simulink model "SimControl_new"  (R2021b)
settings: Solver=ode45  StartTime=0.0  StopTime=inf  RelTol=1e-3
libraries: slpidlib x3, etargetslib x2, dspnetwork x2, sldrtlib x2, simulink_extras x1
settings Model: Creator=Flight Test Lab  LastModifiedBy=jakub
settings SolverCC: AlgebraicLoopSolver=TrustRegion
settings DataIOCC: SaveFormat=StructureWithTime  ReturnWorkspaceOutputs=off
settings OptimizationCC: LifeSpan=inf
settings DebuggingCC: SFExecutionAtInitializationDiag=none  SFMachineParentedDataDiag=warning  ArithmeticOperatorsInVariantConditions=warning
settings HardwareCC: ProdBitPerSizeT=32  ProdBitPerPtrDiffT=32  ProdWordSize=32  ProdHWDeviceType=Specified
settings SFSimCC: SimUseLocalCustomCode=off  CustomCodeUndefinedFunction=UseInterfaceOnly
settings RTWCC: RTWUseLocalCustomCode=off
settings CodeAppCC: StateflowObjectComments=on

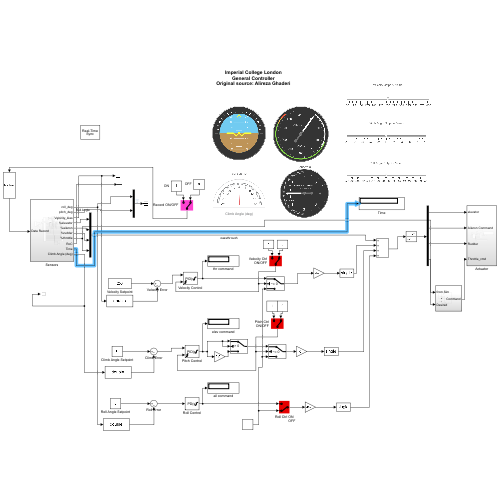
[thumbnail: Simulink's stored preview of the top-level diagram]
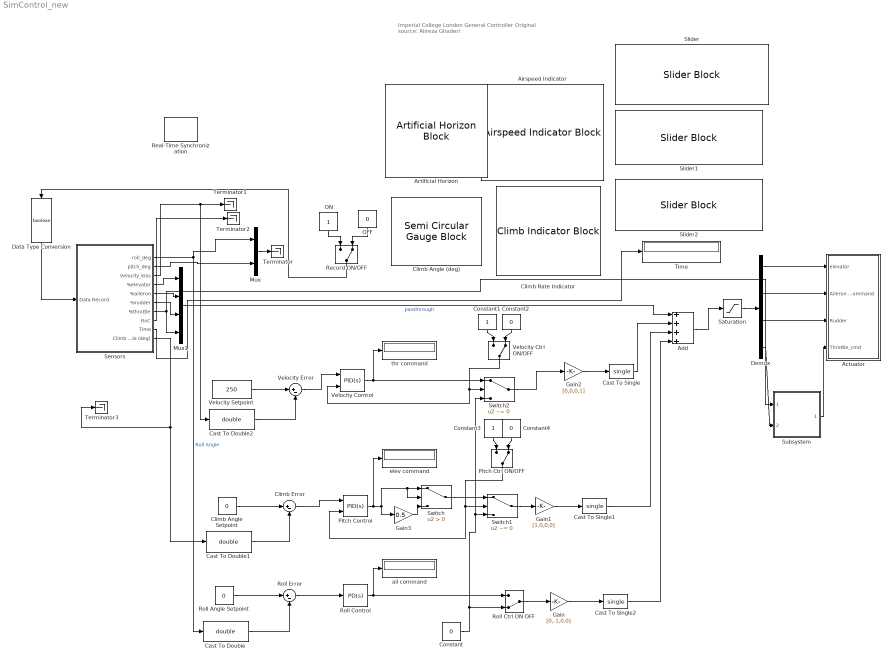
== system SimControl_new ==
  note: Imperial College London
      | General Controller
      | Original source: Alireza Ghaderi
  Actuator : Subsystem
  Add : Sum  Inputs=++++
  Airspeed Indicator : AirspeedIndicatorBlock  LabelPosition=Hide  ScaleMin=0  ScaleMax=450
  Artificial Horizon : ArtificialHorizonBlock  LabelPosition=Hide
  Cast To Double : DataTypeConversion  OutDataTypeStr=double
  Cast To Double1 : DataTypeConversion  OutDataTypeStr=double
  Cast To Double2 : DataTypeConversion  OutDataTypeStr=double
  Cast To Single : DataTypeConversion  OutDataTypeStr=single
  Cast To Single1 : DataTypeConversion  OutDataTypeStr=single
  Cast To Single2 : DataTypeConversion  OutDataTypeStr=single
  Climb Angle (deg) : SemiCircularGaugeBlock  ScaleMin=-20  ScaleMax=20
  Climb Angle Setpoint : Constant  Value=0
  Climb Error : Sum  Inputs=|+-
  Climb Rate Indicator : ClimbIndicatorBlock
  Constant : Constant  Value=0
  Constant1 : Constant
  Constant2 : Constant  Value=0
  Constant3 : Constant
  Constant4 : Constant  Value=0
  Data Type Conversion : DataTypeConversion  OutDataTypeStr=boolean
  Demux : Demux
  Gain : Gain  Gain=[0,-1,0,0]
  Gain1 : Gain  Gain=[1,0,0,0]
  Gain2 : Gain  Gain=[0,0,0,1]
  Gain3 : Gain  Gain=0.5
  Mux : Mux  Inputs=2
  Mux1 : Mux
  OFF : Constant  Value=0
  ON : Constant
  Pitch Control : slpidlib/PID Controller  Controller=PID  Form=Parallel  TimeDomain=Continuous-time  UseExternalTs=off  SampleTime=-1  IntegratorMethod=Forward Euler  FilterMethod=Forward Euler  ControllerParametersSource=internal  P=0.15  I=0.04  D=0.05  UseFilter=on  N=100  TunerSelectOption=Transfer Function Based (PID Tuner App)  InitialConditionSource=internal  InitialConditionForIntegrator=0  InitialConditionForFilter=0  DifferentiatorICPrevScaledInput=0  ExternalReset=rising  TrackingMode=off  Kt=1  LimitOutput=on  SatLimitsSource=internal  UpperSaturationLimit=1  LowerSaturationLimit=-2  LinearizeAsGain=on  AntiWindupMode=clamping  Kb=1  POutMin=[]  POutMax=[]  IOutMin=[]  IOutMax=[]  DOutMin=[]  DOutMax=[]  NOutMin=[]  NOutMax=[]  SumOutMin=[]  SumOutMax=[]  SaturationOutMin=[]  SaturationOutMax=[]  PParamMin=[]  PParamMax=[]  IParamMin=[]  IParamMax=[]  DParamMin=[]  DParamMax=[]  NParamMin=[]  NParamMax=[]  KbParamMin=[]  KbParamMax=[]  KtParamMin=[]  KtParamMax=[]  KbOutMin=[]  KbOutMax=[]  KtOutMin=[]  KtOutMax=[]  IntegratorOutMin=[]  IntegratorOutMax=[]  FilterOutMin=[]  FilterOutMax=[]  SumI1OutMin=[]  SumI1OutMax=[]  SumI2OutMin=[]  SumI2OutMax=[]  SumI3OutMin=[]  SumI3OutMax=[]  SumI4OutMin=[]  SumI4OutMax=[]  SumDOutMin=[]  SumDOutMax=[]  DifferentiatorOutMin=[]  DifferentiatorOutMax=[]  FilterDiffOutCoefMin=[]  FilterDiffOutCoefMax=[]  ReciprocalOutMin=[]  ReciprocalOutMax=[]  SumDenOutMin=[]  SumDenOutMax=[]  SumNumOutMin=[]  SumNumOutMax=[]  DivideOutMin=[]  DivideOutMax=[]  UdiffTsProdOutMin=[]  UdiffTsProdOutMax=[]  NTsProdOutMin=[]  NTsProdOutMax=[]  UintegralTsProdOutMin=[]  UintegralTsProdOutMax=[]  UngainTsProdOutMin=[]  UngainTsProdOutMax=[]  IntegratorContinuousStateAttributes=''  IntegratorStateMustResolveToSignalObject=off  IntegratorRTWStateStorageClass=Auto  FilterContinuousStateAttributes=''  FilterStateMustResolveToSignalObject=off  FilterRTWStateStorageClass=Auto  ParallelPVariant=InternalParameters  IdealPVariant=Disabled  IVariant=InternalParameters  DVariant=InternalParameters  IntegratorVariant=Continuous  SatVariant=Enabled  AWVariant=ContClampingParallel  PCopyVariant=Disabled  TRVariant=Disabled  FdbkBlocksVariant=Forward  IdealPFdbkVariant=Disabled  SatFdbkVariant=Disabled  DerivativeFilterVariant=ContFilter  NVariant=InternalParameters  NCopyVariant=Disabled  FilterICVariant=InternalICsFilter  IntegratorICVariant=InternalICs  ExternalResetVariant=ExternalReset  TRSumVariant=Passthrough  SumFdbkVariant=Disabled  SumVariant=Sum_PID  TsampFilterVariant=InternalTs  TsampNgainVariant=Passthrough  TsampIntegralVariant=Passthrough  ExternalSaturationOutDataTypeStr=Inherit: Same as second input
  Pitch Ctrl ON/OFF : ManualSwitch  CurrentSetting=0
  Real-Time Synchronization : sldrtlib/Real-Time Synchronization  SampleTime=0.05  MaxMissedTicks=100  ShowMissedTicks=off  YieldWhenWaiting=off
  Record ON/OFF : ManualSwitch  CurrentSetting=0
  Roll Angle Setpoint : Constant  Value=0
  Roll Control : slpidlib/PID Controller  Controller=PD  Form=Parallel  TimeDomain=Continuous-time  UseExternalTs=off  SampleTime=-1  IntegratorMethod=Forward Euler  FilterMethod=Forward Euler  ControllerParametersSource=internal  P=-0.7  I=1  D=-0.05  UseFilter=on  N=100  TunerSelectOption=Transfer Function Based (PID Tuner App)  InitialConditionSource=internal  InitialConditionForIntegrator=0  InitialConditionForFilter=0  DifferentiatorICPrevScaledInput=0  ExternalReset=none  TrackingMode=off  Kt=1  LimitOutput=on  SatLimitsSource=internal  UpperSaturationLimit=1  LowerSaturationLimit=-1  LinearizeAsGain=on  AntiWindupMode=none  Kb=1  POutMin=[]  POutMax=[]  IOutMin=[]  IOutMax=[]  DOutMin=[]  DOutMax=[]  NOutMin=[]  NOutMax=[]  SumOutMin=[]  SumOutMax=[]  SaturationOutMin=[]  SaturationOutMax=[]  PParamMin=[]  PParamMax=[]  IParamMin=[]  IParamMax=[]  DParamMin=[]  DParamMax=[]  NParamMin=[]  NParamMax=[]  KbParamMin=[]  KbParamMax=[]  KtParamMin=[]  KtParamMax=[]  KbOutMin=[]  KbOutMax=[]  KtOutMin=[]  KtOutMax=[]  IntegratorOutMin=[]  IntegratorOutMax=[]  FilterOutMin=[]  FilterOutMax=[]  SumI1OutMin=[]  SumI1OutMax=[]  SumI2OutMin=[]  SumI2OutMax=[]  SumI3OutMin=[]  SumI3OutMax=[]  SumI4OutMin=[]  SumI4OutMax=[]  SumDOutMin=[]  SumDOutMax=[]  DifferentiatorOutMin=[]  DifferentiatorOutMax=[]  FilterDiffOutCoefMin=[]  FilterDiffOutCoefMax=[]  ReciprocalOutMin=[]  ReciprocalOutMax=[]  SumDenOutMin=[]  SumDenOutMax=[]  SumNumOutMin=[]  SumNumOutMax=[]  DivideOutMin=[]  DivideOutMax=[]  UdiffTsProdOutMin=[]  UdiffTsProdOutMax=[]  NTsProdOutMin=[]  NTsProdOutMax=[]  UintegralTsProdOutMin=[]  UintegralTsProdOutMax=[]  UngainTsProdOutMin=[]  UngainTsProdOutMax=[]  IntegratorContinuousStateAttributes=''  IntegratorStateMustResolveToSignalObject=off  IntegratorRTWStateStorageClass=Auto  FilterContinuousStateAttributes=''  FilterStateMustResolveToSignalObject=off  FilterRTWStateStorageClass=Auto  ParallelPVariant=InternalParameters  IdealPVariant=Disabled  IVariant=Disabled  DVariant=InternalParameters  IntegratorVariant=Disabled  SatVariant=Enabled  AWVariant=Disabled  PCopyVariant=Disabled  TRVariant=Disabled  FdbkBlocksVariant=Forward  IdealPFdbkVariant=Disabled  SatFdbkVariant=Disabled  DerivativeFilterVariant=ContFilter  NVariant=InternalParameters  NCopyVariant=Disabled  FilterICVariant=InternalICsFilter  IntegratorICVariant=Disabled  ExternalResetVariant=Disabled  TRSumVariant=Passthrough  SumFdbkVariant=Disabled  SumVariant=Sum_PD  TsampFilterVariant=InternalTs  TsampNgainVariant=Passthrough  TsampIntegralVariant=Disabled_SignalSpec  ExternalSaturationOutDataTypeStr=Inherit: Same as second input
  Roll Ctrl ON OFF : ManualSwitch  CurrentSetting=0
  Roll Error : Sum  Inputs=|+-
  Saturation : Saturate  UpperLimit=[1,1,1,1]  LowerLimit=[-1,-1,-1,0]
  Sensors : Subsystem
  Slider : SliderBlock  ScaleMin=100  ScaleMax=400
  Slider1 : SliderBlock  ScaleMin=-10  ScaleMax=10  TickInterval=2
  Slider2 : SliderBlock  ScaleMin=-45  ScaleMax=45
  Subsystem : Subsystem
  Switch : Switch  Criteria=u2 > Threshold
  Switch1 : Switch  Criteria=u2 ~= 0
  Switch2 : Switch  Criteria=u2 ~= 0
  Terminator{,1..3} (4 alike) : Terminator
  Time : Display
  Velocity Control : slpidlib/PID Controller  Controller=PID  Form=Parallel  TimeDomain=Continuous-time  UseExternalTs=off  SampleTime=-1  IntegratorMethod=Forward Euler  FilterMethod=Forward Euler  ControllerParametersSource=internal  P=3  I=0.1  D=0.2  UseFilter=on  N=100  TunerSelectOption=Transfer Function Based (PID Tuner App)  InitialConditionSource=internal  InitialConditionForIntegrator=0  InitialConditionForFilter=0  DifferentiatorICPrevScaledInput=0  ExternalReset=rising  TrackingMode=off  Kt=1  LimitOutput=on  SatLimitsSource=internal  UpperSaturationLimit=1  LowerSaturationLimit=-1  LinearizeAsGain=on  AntiWindupMode=clamping  Kb=1  POutMin=[]  POutMax=[]  IOutMin=[]  IOutMax=[]  DOutMin=[]  DOutMax=[]  NOutMin=[]  NOutMax=[]  SumOutMin=[]  SumOutMax=[]  SaturationOutMin=[]  SaturationOutMax=[]  PParamMin=[]  PParamMax=[]  IParamMin=[]  IParamMax=[]  DParamMin=[]  DParamMax=[]  NParamMin=[]  NParamMax=[]  KbParamMin=[]  KbParamMax=[]  KtParamMin=[]  KtParamMax=[]  KbOutMin=[]  KbOutMax=[]  KtOutMin=[]  KtOutMax=[]  IntegratorOutMin=[]  IntegratorOutMax=[]  FilterOutMin=[]  FilterOutMax=[]  SumI1OutMin=[]  SumI1OutMax=[]  SumI2OutMin=[]  SumI2OutMax=[]  SumI3OutMin=[]  SumI3OutMax=[]  SumI4OutMin=[]  SumI4OutMax=[]  SumDOutMin=[]  SumDOutMax=[]  DifferentiatorOutMin=[]  DifferentiatorOutMax=[]  FilterDiffOutCoefMin=[]  FilterDiffOutCoefMax=[]  ReciprocalOutMin=[]  ReciprocalOutMax=[]  SumDenOutMin=[]  SumDenOutMax=[]  SumNumOutMin=[]  SumNumOutMax=[]  DivideOutMin=[]  DivideOutMax=[]  UdiffTsProdOutMin=[]  UdiffTsProdOutMax=[]  NTsProdOutMin=[]  NTsProdOutMax=[]  UintegralTsProdOutMin=[]  UintegralTsProdOutMax=[]  UngainTsProdOutMin=[]  UngainTsProdOutMax=[]  IntegratorContinuousStateAttributes=''  IntegratorStateMustResolveToSignalObject=off  IntegratorRTWStateStorageClass=Auto  FilterContinuousStateAttributes=''  FilterStateMustResolveToSignalObject=off  FilterRTWStateStorageClass=Auto  ParallelPVariant=InternalParameters  IdealPVariant=Disabled  IVariant=InternalParameters  DVariant=InternalParameters  IntegratorVariant=Continuous  SatVariant=Enabled  AWVariant=ContClampingParallel  PCopyVariant=Disabled  TRVariant=Disabled  FdbkBlocksVariant=Forward  IdealPFdbkVariant=Disabled  SatFdbkVariant=Disabled  DerivativeFilterVariant=ContFilter  NVariant=InternalParameters  NCopyVariant=Disabled  FilterICVariant=InternalICsFilter  IntegratorICVariant=InternalICs  ExternalResetVariant=ExternalReset  TRSumVariant=Passthrough  SumFdbkVariant=Disabled  SumVariant=Sum_PID  TsampFilterVariant=InternalTs  TsampNgainVariant=Passthrough  TsampIntegralVariant=Passthrough  ExternalSaturationOutDataTypeStr=Inherit: Same as second input
  Velocity Ctrl ON/OFF : ManualSwitch  CurrentSetting=0
  Velocity Error : Sum  Inputs=|+-
  Velocity Setpoint : Constant  Value=250
  ail command : Display
  elev command : Display
  thr command : Display
  wires:
  Sensors/1(roll_deg) -> Mux/1, Cast To Double/1  "Roll Angle"
  Sensors/2(pitch_deg) -> Mux/2
  Mux/1 -> Terminator/1
  Sensors/4(%elevator) -> Mux1/1
  Sensors/5(%aileron) -> Mux1/2
  Sensors/6(%rudder) -> Mux1/3
  Sensors/7(%throttle) -> Mux1/4, Subsystem/1(from Sim)
  Demux/1 -> Actuator/1(elevator)
  Demux/2 -> Actuator/2(Aileron Command)
  Demux/3 -> Actuator/3("Rudder ")
  Sensors/3(Velocity_kias) -> Terminator1/1, Cast To Double2/1
  Mux1/1 -> Add/1  "passthrough"
  Roll Angle Setpoint/1 -> Roll Error/1
  Climb Angle Setpoint/1 -> Climb Error/1
  Velocity Setpoint/1 -> Velocity Error/1
  Roll Ctrl ON OFF/1 -> Gain/1
  Gain/1 -> Cast To Single2/1
  Constant/1 -> Roll Ctrl ON OFF/2, Switch2/3, Switch1/3
  Roll Error/1 -> Roll Control/1
  Roll Control/1 -> ail command/1, Roll Ctrl ON OFF/1
  Cast To Double/1 -> Roll Error/2
  Cast To Double1/1 -> Climb Error/2
  Cast To Double2/1 -> Velocity Error/2
  Velocity Error/1 -> Velocity Control/1
  Climb Error/1 -> Pitch Control/1
  Gain1/1 -> Cast To Single1/1
  Switch1/1 -> Gain1/1
  Gain3/1 -> Switch/3
  Pitch Control/1 -> elev command/1, Gain3/1, Switch/1, Switch/2
  Switch/1 -> Switch1/1
  Add/1 -> Saturation/1
  Saturation/1 -> Demux/1
  Velocity Control/1 -> thr command/1, Switch2/1
  Cast To Single/1 -> Add/2
  Cast To Single1/1 -> Add/3
  Cast To Single2/1 -> Add/4
  Record ON/OFF/1 -> Data Type Conversion/1
  OFF/1 -> Record ON/OFF/2
  ON/1 -> Record ON/OFF/1
  Data Type Conversion/1 -> Sensors/1(Data Record)
  Sensors/8(RoC) -> Terminator2/1
  Sensors/9(Time) -> Time/1
  Sensors/10(Climb Angle (deg)) -> Terminator3/1, Cast To Double1/1
  Velocity Ctrl ON/OFF/1 -> Switch2/2, Velocity Control/2
  Pitch Ctrl ON/OFF/1 -> Pitch Control/2, Switch1/2
  Constant1/1 -> Velocity Ctrl ON/OFF/1
  Constant2/1 -> Velocity Ctrl ON/OFF/2
  Constant3/1 -> Pitch Ctrl ON/OFF/1
  Constant4/1 -> Pitch Ctrl ON/OFF/2
  Subsystem/1(Command) -> Actuator/4(Throttle_cmd)
  Switch2/1 -> Gain2/1
  Gain2/1 -> Cast To Single/1
  Demux/4 -> Subsystem/2(Desired)

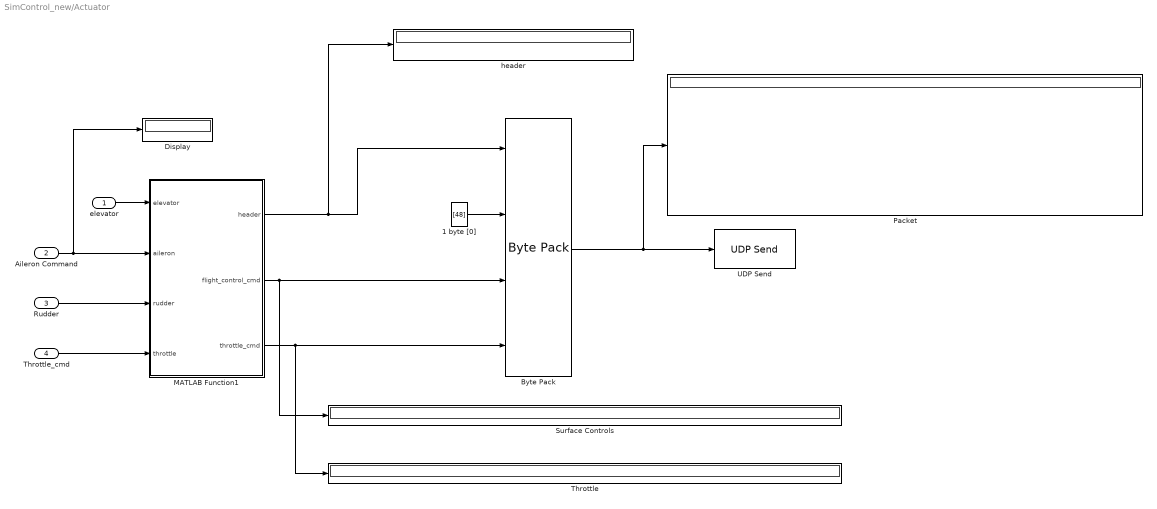
== system SimControl_new/Actuator ==
  elevator : Inport
  Aileron Command : Inport  Port=2
  "Rudder " : Inport  Port=3
  Throttle_cmd : Inport  Port=4
  1 byte [0] : Constant  Value=[48]  OutDataTypeStr=uint8
  Byte Pack : etargetslib/Byte Pack  datatypes={'uint8','uint8','single','single'}  byteAlign=1
  Display : Display
  MATLAB Function1 : MATLAB Function  TreatAsAtomicUnit=on
  Packet : Display
  Surface Controls : Display
  Throttle : Display
  UDP Send : dspnetwork/UDP Send  remoteURL='192.168.5.211'  remotePort=49000  localURL='0.0.0.0'  localPortSource=Automatically determine  localPort=-1  sendBufferSize=8192  sampletime=-1  blockPlatform=[]  separateLengthPort=0
  header : Display
  wires:
  MATLAB Function1/2(flight_control_cmd) -> Surface Controls/1, Byte Pack/3
  Byte Pack/1 -> UDP Send/1, Packet/1
  MATLAB Function1/3(throttle_cmd) -> Throttle/1, Byte Pack/4
  MATLAB Function1/1(header) -> Byte Pack/1, header/1
  elevator/1 -> MATLAB Function1/1(elevator)
  1 byte [0]/1 -> Byte Pack/2
  Throttle_cmd/1 -> MATLAB Function1/4(throttle)
  "Rudder "/1 -> MATLAB Function1/3(rudder)
  Aileron Command/1 -> MATLAB Function1/2(aileron), Display/1

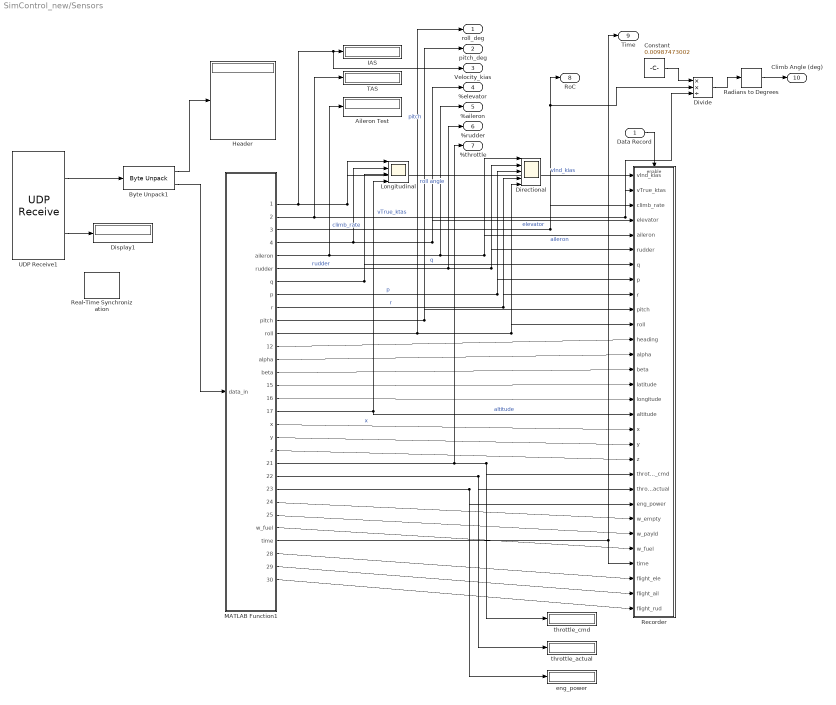
== system SimControl_new/Sensors ==
  Data Record : Inport
  Aileron Test : Display
  Byte Unpack1 : etargetslib/Byte Unpack  dimensions={5,[9,15]}  datatypes={'uint8','single'}  byteAlign=1
  Constant : Constant  Value=0.00987473002
  Directional : Scope  NumInputPorts=5
  Display1 : Display
  Divide : Product  Inputs=**/
  Header : Display
  IAS : Display
  Longitudinal : Scope  NumInputPorts=4
  MATLAB Function1 : MATLAB Function  TreatAsAtomicUnit=on
  Radians to Degrees : simulink_extras/Transformations/Radians to Degrees
  Real-Time Synchronization : sldrtlib/Real-Time Synchronization  SampleTime=0.0125  MaxMissedTicks=1000  ShowMissedTicks=off  YieldWhenWaiting=off
  Recorder : Subsystem
  TAS : Display
  UDP Receive1 : dspnetwork/UDP Receive  localURL='0.0.0.0'  localPort=49300  remoteURL='192.168.5.211'  remotePort=-1  recvBufferSize=8192  dims=545  signalDatatype=uint8  isComplex=off  isVarSize=off  showBlockingTime=off  blockingTime=0  sampletime=0.0125  blockPlatform=[]
  eng_power : Display
  throttle_actual : Display
  throttle_cmd : Display
  roll_deg : Outport
  pitch_deg : Outport  Port=2
  Velocity_kias : Outport  Port=3
  %elevator : Outport  Port=4
  %aileron : Outport  Port=5
  %rudder : Outport  Port=6
  %throttle : Outport  Port=7
  RoC : Outport  Port=8
  Time : Outport  Port=9
  Climb Angle (deg) : Outport  Port=10
  wires:
  MATLAB Function1/3(climb_rate) -> RoC/1, Divide/2, Recorder/3(climb_rate)  "climb_rate"
  MATLAB Function1/1(vInd_kias) -> Velocity_kias/1, IAS/1, Longitudinal/1, Recorder/1(vInd_kias)  "vInd_kias"
  MATLAB Function1/21(throttle_cmd) -> throttle_cmd/1, Recorder/21(throttle_cmd), %throttle/1
  MATLAB Function1/22(throttle_actual) -> throttle_actual/1, Recorder/22(throttle_actual)
  MATLAB Function1/15(latitutde) -> Recorder/15(latitude)
  MATLAB Function1/25(w_payld) -> Recorder/25(w_payld)
  MATLAB Function1/11(roll) -> roll_deg/1, Directional/5, Recorder/11(roll)  "roll angle"
  MATLAB Function1/8(p) -> Recorder/8(p), Directional/3  "p"
  MATLAB Function1/18(x) -> Recorder/18(x)  "x"
  MATLAB Function1/5(aileron) -> Aileron Test/1, Directional/1, Recorder/5(aileron), %aileron/1  "aileron"
  MATLAB Function1/6(rudder) -> Recorder/6(rudder), Directional/2, %rudder/1  "rudder"
  MATLAB Function1/14(beta) -> Recorder/14(beta)
  MATLAB Function1/12(heading_true) -> Recorder/12(heading)
  MATLAB Function1/2(vTrue_ktas) -> TAS/1, Divide/3, Recorder/2(vTrue_ktas)  "vTrue_ktas"
  MATLAB Function1/17(altitude) -> Longitudinal/4, Recorder/17(altitude)  "altitude"
  MATLAB Function1/19(y) -> Recorder/19(y)
  Byte Unpack1/1 -> Header/1
  MATLAB Function1/20(z) -> Recorder/20(z)
  MATLAB Function1/23(eng_power) -> eng_power/1, Recorder/23(eng_power)
  MATLAB Function1/4(elevator) -> Longitudinal/2, Recorder/4(elevator), %elevator/1  "elevator"
  UDP Receive1/2 -> Display1/1
  MATLAB Function1/26(w_fuel) -> Recorder/26(w_fuel)
  MATLAB Function1/9(r) -> Directional/4, Recorder/9(r)  "r"
  MATLAB Function1/10(pitch) -> pitch_deg/1, Recorder/10(pitch)  "pitch"
  Byte Unpack1/2 -> MATLAB Function1/1(data_in)
  UDP Receive1/1 -> Byte Unpack1/1
  MATLAB Function1/24(w_empty) -> Recorder/24(w_empty)
  MATLAB Function1/30(flight_rud) -> Recorder/30(flight_rud)
  MATLAB Function1/29(flight_ail) -> Recorder/29(flight_ail)
  MATLAB Function1/27(time) -> Time/1, Recorder/27(time)
  MATLAB Function1/28(flight_ele) -> Recorder/28(flight_ele)
  MATLAB Function1/16(longitude) -> Recorder/16(longitude)
  Data Record/1 -> Recorder/Enable
  MATLAB Function1/7(q) -> Longitudinal/3, Recorder/7(q)  "q"
  MATLAB Function1/13(alpha) -> Recorder/13(alpha)
  Constant/1 -> Divide/1
  Divide/1 -> Radians to Degrees/1
  Radians to Degrees/1 -> Climb Angle (deg)/1

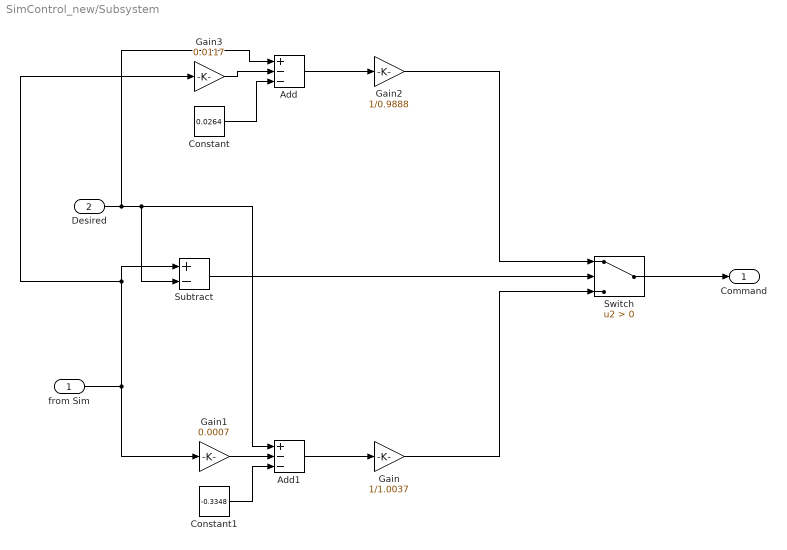
== system SimControl_new/Subsystem ==
  from Sim : Inport
  Desired : Inport  Port=2
  Add : Sum  Inputs=+--
  Add1 : Sum  Inputs=+--
  Constant : Constant  Value=0.0264
  Constant1 : Constant  Value=-0.3348
  Gain : Gain  Gain=1/1.0037
  Gain1 : Gain  Gain=0.0007
  Gain2 : Gain  Gain=1/0.9888
  Gain3 : Gain  Gain=0.0117
  Subtract : Sum  Inputs=+-
  Switch : Switch  Criteria=u2 > Threshold
  Command : Outport
  wires:
  Switch/1 -> Command/1
  Subtract/1 -> Switch/2
  from Sim/1 -> Gain1/1, Subtract/1, Gain3/1
  Gain3/1 -> Add/2
  Constant/1 -> Add/3
  Gain1/1 -> Add1/2
  Desired/1 -> Subtract/2, Add1/1, Add/1
  Constant1/1 -> Add1/3
  Add/1 -> Gain2/1
  Add1/1 -> Gain/1
  Gain/1 -> Switch/3
  Gain2/1 -> Switch/1

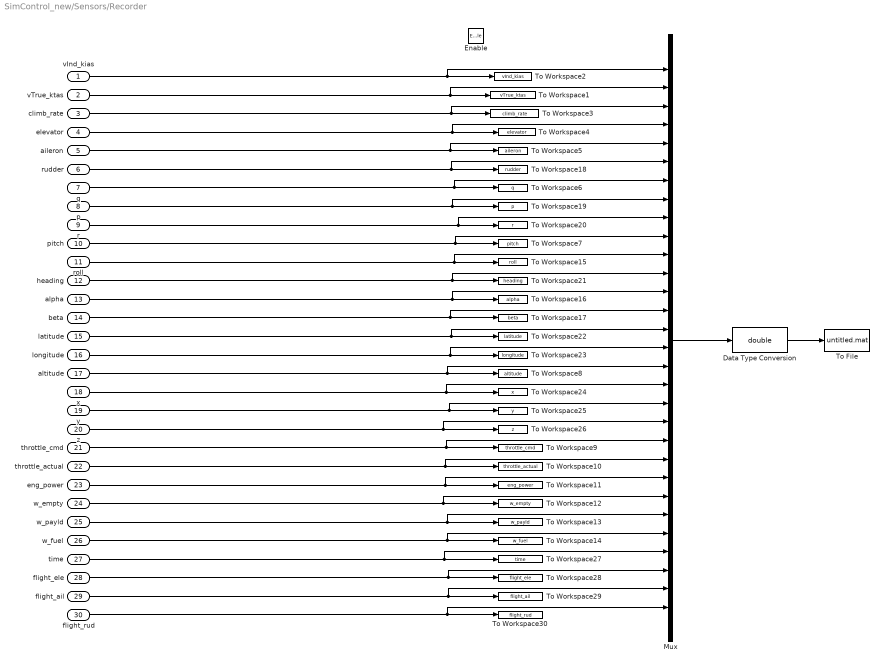
== system SimControl_new/Sensors/Recorder ==
  vInd_kias : Inport
  vTrue_ktas : Inport  Port=2
  climb_rate : Inport  Port=3
  elevator : Inport  Port=4
  aileron : Inport  Port=5
  rudder : Inport  Port=6
  q : Inport  Port=7
  p : Inport  Port=8
  r : Inport  Port=9
  pitch : Inport  Port=10
  roll : Inport  Port=11
  heading : Inport  Port=12
  alpha : Inport  Port=13
  beta : Inport  Port=14
  latitude : Inport  Port=15
  longitude : Inport  Port=16
  altitude : Inport  Port=17
  x : Inport  Port=18
  y : Inport  Port=19
  z : Inport  Port=20
  throttle_cmd : Inport  Port=21
  throttle_actual : Inport  Port=22
  eng_power : Inport  Port=23
  w_empty : Inport  Port=24
  w_payld : Inport  Port=25
  w_fuel : Inport  Port=26
  time : Inport  Port=27
  flight_ele : Inport  Port=28
  flight_ail : Inport  Port=29
  flight_rud : Inport  Port=30
  Enable : EnablePort
  Data Type Conversion : DataTypeConversion  OutDataTypeStr=double
  Mux : Mux  Inputs=30
  To File : ToFile  MatrixName=data  SaveFormat=Timeseries
  To Workspace1 : ToWorkspace  VariableName=vTrue_ktas  SampleTime=-1
  To Workspace10 : ToWorkspace  VariableName=throttle_actual  SampleTime=-1
  To Workspace11 : ToWorkspace  VariableName=eng_power  SampleTime=-1
  To Workspace12 : ToWorkspace  VariableName=w_empty  SampleTime=-1
  To Workspace13 : ToWorkspace  VariableName=w_payld  SampleTime=-1
  To Workspace14 : ToWorkspace  VariableName=w_fuel  SampleTime=-1
  To Workspace15 : ToWorkspace  VariableName=roll  SampleTime=-1
  To Workspace16 : ToWorkspace  VariableName=alpha  SampleTime=-1
  To Workspace17 : ToWorkspace  VariableName=beta  SampleTime=-1
  To Workspace18 : ToWorkspace  VariableName=rudder  SampleTime=-1
  To Workspace19 : ToWorkspace  VariableName=p  SampleTime=-1
  To Workspace2 : ToWorkspace  VariableName=vInd_kias  SampleTime=-1
  To Workspace20 : ToWorkspace  VariableName=r  SampleTime=-1
  To Workspace21 : ToWorkspace  VariableName=heading  SampleTime=-1
  To Workspace22 : ToWorkspace  VariableName=latitude  SampleTime=-1
  To Workspace23 : ToWorkspace  VariableName=longitude  SampleTime=-1
  To Workspace24 : ToWorkspace  VariableName=x  SampleTime=-1
  To Workspace25 : ToWorkspace  VariableName=y  SampleTime=-1
  To Workspace26 : ToWorkspace  VariableName=z  SampleTime=-1
  To Workspace27 : ToWorkspace  VariableName=time  SampleTime=-1
  To Workspace28 : ToWorkspace  VariableName=flight_ele  SampleTime=-1
  To Workspace29 : ToWorkspace  VariableName=flight_ail  SampleTime=-1
  To Workspace3 : ToWorkspace  VariableName=climb_rate  SampleTime=-1
  To Workspace30 : ToWorkspace  VariableName=flight_rud  SampleTime=-1
  To Workspace4 : ToWorkspace  VariableName=elevator  SampleTime=-1
  To Workspace5 : ToWorkspace  VariableName=aileron  SampleTime=-1
  To Workspace6 : ToWorkspace  VariableName=q  SampleTime=-1
  To Workspace7 : ToWorkspace  VariableName=pitch  SampleTime=-1
  To Workspace8 : ToWorkspace  VariableName=altitude  SampleTime=-1
  To Workspace9 : ToWorkspace  VariableName=throttle_cmd  SampleTime=-1
  wires:
  pitch/1 -> Mux/10, To Workspace7/1
  z/1 -> Mux/20, To Workspace26/1
  q/1 -> Mux/7, To Workspace6/1
  vInd_kias/1 -> Mux/1, To Workspace2/1
  beta/1 -> Mux/14, To Workspace17/1
  longitude/1 -> Mux/16, To Workspace23/1
  climb_rate/1 -> Mux/3, To Workspace3/1
  vTrue_ktas/1 -> Mux/2, To Workspace1/1
  heading/1 -> Mux/12, To Workspace21/1
  w_fuel/1 -> Mux/26, To Workspace14/1
  r/1 -> Mux/9, To Workspace20/1
  w_payld/1 -> Mux/25, To Workspace13/1
  altitude/1 -> Mux/17, To Workspace8/1
  aileron/1 -> Mux/5, To Workspace5/1
  w_empty/1 -> Mux/24, To Workspace12/1
  alpha/1 -> Mux/13, To Workspace16/1
  p/1 -> Mux/8, To Workspace19/1
  throttle_cmd/1 -> Mux/21, To Workspace9/1
  rudder/1 -> Mux/6, To Workspace18/1
  eng_power/1 -> Mux/23, To Workspace11/1
  elevator/1 -> Mux/4, To Workspace4/1
  roll/1 -> Mux/11, To Workspace15/1
  throttle_actual/1 -> Mux/22, To Workspace10/1
  y/1 -> Mux/19, To Workspace25/1
  latitude/1 -> Mux/15, To Workspace22/1
  x/1 -> Mux/18, To Workspace24/1
  time/1 -> Mux/27, To Workspace27/1
  flight_ele/1 -> Mux/28, To Workspace28/1
  flight_ail/1 -> Mux/29, To Workspace29/1
  flight_rud/1 -> Mux/30, To Workspace30/1
  Mux/1 -> Data Type Conversion/1
  Data Type Conversion/1 -> To File/1

== matlab function SimControl_new/Actuator/MATLAB Function1 ==
  data: elevator input; header output uint8; flight_control_cmd output; aileron input single; rudder input single; throttle input; throttle_cmd output single
function [header,flight_control_cmd,throttle_cmd] = fcn(elevator, aileron, rudder, throttle) 
header =[uint8(68) uint8(65) uint8(84) uint8(65)];
No_Comand = single(-999);
 %Surface_header = typecast(uint8([uint8(8) uint8(0) uint8(0) uint8(0)]),'single')
%surfaces_control_cmd = [1.1210388e-44 elevator aileron rudder No_Comand No_Comand No_Comand No_Comand No_Comand  ];
%Flight_Control_Surface_header = typecast(uint8([uint8(11) uint8(0) uint8(0) uint8(0)]),'single')
flight_control_cmd = [1.541428310757299e-44 elevator aileron rudder No_Comand No_Comand No_Comand No_Comand No_Comand  ];
%Throttle_header = typecast(uint8([uint8(25) uint8(0) uint8(0) uint8(0)]),'single');
%throttle_cmd = [3.503246160812043e-44 throttle throttle No_Comand No_Comand No_Comand No_Comand No_Comand No_Comand];
throttle_cmd = [3.64337600724e-44 throttle throttle No_Comand No_Comand No_Comand No_Comand No_Comand No_Comand];
end

== matlab function SimControl_new/Sensors/MATLAB Function1 ==
  data: vInd_kias output; vTrue_ktas output; climb_rate output; elevator output; aileron output; rudder output; q output; p output; r output; pitch output; roll output; heading_true output; alpha output; beta output; latitutde output; longitude output; altitude output; x output; y output; z output; throttle_cmd output; throttle_actual output; eng_power output; w_empty output; w_payld output; w_fuel output; time output; data_in input; flight_ele output; flight_ail output; flight_rud output
function [vInd_kias,vTrue_ktas,...
    climb_rate,...
    elevator,aileron,rudder,...
    q,p,r,...
    pitch, roll, heading_true,...
    alpha,beta,...
    latitutde, longitude, altitude,...
    x,y,z,...
    throttle_cmd,...
    throttle_actual,...
    eng_power,...
    w_empty,w_payld,w_fuel,...
    time,...
    flight_ele,flight_ail,flight_rud] = decoder(data_in)
 frame_rate = data_in(2,1);
 time = data_in(2,2);
 vInd_kias = data_in(2,3);
 vTrue_ktas = data_in(4,3);
 climb_rate = data_in(4,4);
 elevator = data_in(2,5); %Joystick elevator value
 aileron = data_in(3,5);  %Joystick aileron value
 rudder= data_in(4,5);    %Joystick rudder value
 flight_ele = data_in(2,6);
 flight_ail = data_in(3,6);
 flight_rud = data_in(4,6);
 q= data_in(2,7);
 p= data_in(3,7);
 r= data_in(4,7);
 pitch= data_in(2,8);
 roll= data_in(3,8);
 heading_true= data_in(4,8);
 alpha = data_in(2,9);
 beta  = data_in(3,9);
 latitutde= data_in(2,10);
 longitude= data_in(3,10);
 altitude= data_in(4,10);
 x = data_in(2,11);
 y = data_in(3,11);
 z = data_in(4,11);
 throttle_cmd = data_in(2,12);
 throttle_actual = data_in(2,13);
 eng_power = data_in(2,14);
 w_empty = data_in(2,15);
 w_payld = data_in(3,15);
 w_fuel  = data_in(4,15);
end
